simulink model "benchmark"  (R2024a)
settings: Solver=FixedStepAuto  StartTime=0.0  StopTime=10.0  FixedStep=0.001  RelTol=1e-3
InitFcn:
  | run("estimators_design.m")
libraries: cstblocks x1
settings Model: Creator=Bocchio  LastModifiedBy=Bocchio

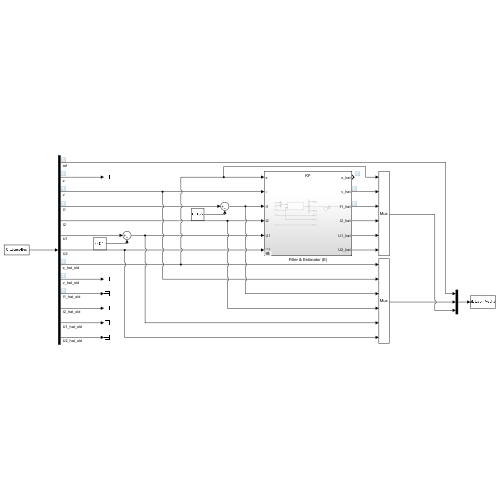
[thumbnail: Simulink's stored preview of the top-level diagram]
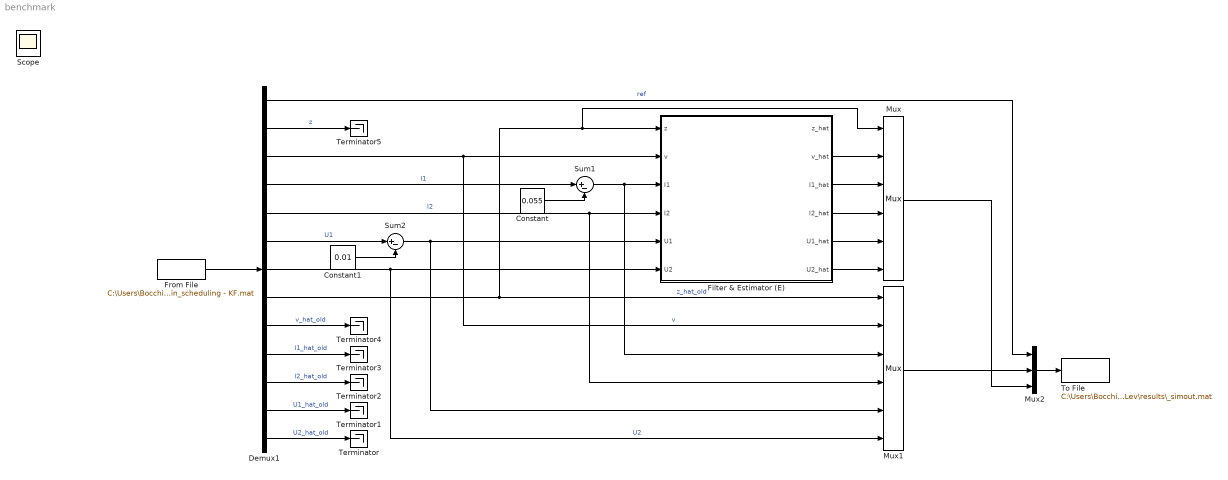
== system benchmark ==
  Constant : Constant  Value=0.055
  Constant1 : Constant  Value=0.01
  Demux1 : Demux  Outputs=13
  Filter & Estimator (E) : Subsystem  Variant=on  VariantControlMode=label  LabelModeActiveChoice=KF
  From File : FromFile  FileName=C:\Users\Bocchio\OneDrive\University\Lab - Mechatronics\MagLev\results\step\PID_gain_scheduling - KF.mat  SampleTime=0.001  InterpolationWithinTimeRange=Zero order hold
  Mux : Mux  Inputs=6
  Mux1 : Mux  Inputs=6
  Mux2 : Mux  Inputs=3
  Sum1 : Sum  Inputs=|+-
  Sum2 : Sum  Inputs=|+-
  Terminator{,1..5} (6 alike) : Terminator
  To File : ToFile  Filename=C:\Users\Bocchio\OneDrive\University\Lab - Mechatronics\MagLev\results\_simout.mat  MatrixName=logouts
  Scope : Scope
  wires:
  From File/1 -> Demux1/1
  Demux1/1 -> Mux2/1  "ref"
  Demux1/2 -> Terminator5/1  "z"
  Demux1/3 -> Mux1/2, Filter & Estimator (E)/2(v)  "v"
  Demux1/5 -> Mux1/4, Filter & Estimator (E)/4(I2)  "I2"
  Demux1/7 -> Filter & Estimator (E)/6(U2), Mux1/6  "U2"
  Demux1/8 -> Mux/1, Filter & Estimator (E)/1(z), Mux1/1  "z_hat_old"
  Demux1/9 -> Terminator4/1  "v_hat_old"
  Demux1/10 -> Terminator3/1  "I1_hat_old"
  Demux1/11 -> Terminator2/1  "I2_hat_old"
  Filter & Estimator (E)/2(v_hat) -> Mux/2
  Filter & Estimator (E)/3(I1_hat) -> Mux/3
  Filter & Estimator (E)/4(I2_hat) -> Mux/4
  Filter & Estimator (E)/5(U1_hat) -> Mux/5
  Filter & Estimator (E)/6(U2_hat) -> Mux/6
  Demux1/12 -> Terminator1/1  "U1_hat_old"
  Demux1/13 -> Terminator/1  "U2_hat_old"
  Mux/1 -> Mux2/3
  Mux2/1 -> To File/1
  Mux1/1 -> Mux2/2
  Constant/1 -> Sum1/2
  Demux1/4 -> Sum1/1  "I1"
  Sum1/1 -> Filter & Estimator (E)/3(I1), Mux1/3
  Constant1/1 -> Sum2/2
  Demux1/6 -> Sum2/1  "U1"
  Sum2/1 -> Mux1/5, Filter & Estimator (E)/5(U1)

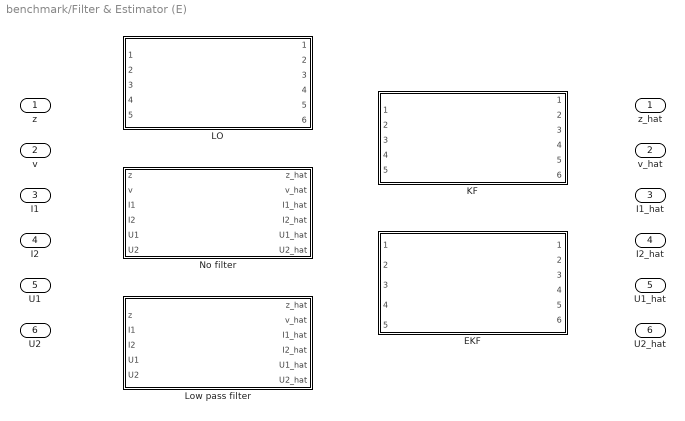
== system benchmark/Filter & Estimator (E) ==
  z : Inport
  v : Inport  Port=2
  I1 : Inport  Port=3
  I2 : Inport  Port=4
  U1 : Inport  Port=5
  U2 : Inport  Port=6
  EKF : Subsystem  VariantControl=EKF  ReferencedSubsystem=EKF
  KF : Subsystem  VariantControl=KF  ReferencedSubsystem=KF
  LO : Subsystem  VariantControl=LO  ReferencedSubsystem=LO
  Low pass filter : Subsystem  VariantControl=Low pass filter
  No filter : Subsystem  VariantControl=No filter
  z_hat : Outport
  v_hat : Outport  Port=2
  I1_hat : Outport  Port=3
  I2_hat : Outport  Port=4
  U1_hat : Outport  Port=5
  U2_hat : Outport  Port=6

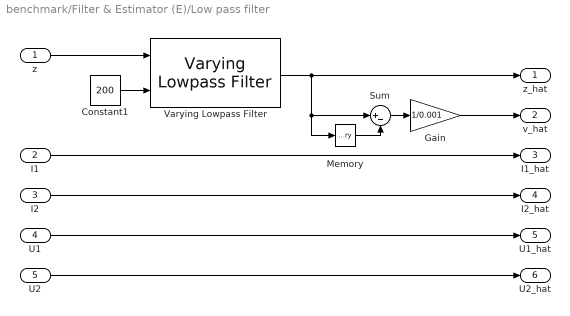
== system benchmark/Filter & Estimator (E)/Low pass filter ==
  z : Inport
  I1 : Inport  Port=2
  I2 : Inport  Port=3
  U1 : Inport  Port=4
  U2 : Inport  Port=5
  Constant1 : Constant  Value=200
  Gain : Gain  Gain=1/0.001
  Memory : Memory
  Sum : Sum  Inputs=|+-
  Varying Lowpass Filter : cstblocks/Linear Parameter Varying/Varying Lowpass Filter  N=1
  z_hat : Outport
  v_hat : Outport  Port=2
  I1_hat : Outport  Port=3
  I2_hat : Outport  Port=4
  U1_hat : Outport  Port=5
  U2_hat : Outport  Port=6
  wires:
  Constant1/1 -> Varying Lowpass Filter/2
  z/1 -> Varying Lowpass Filter/1
  Memory/1 -> Sum/2
  Sum/1 -> Gain/1
  U1/1 -> U1_hat/1
  Varying Lowpass Filter/1 -> Memory/1, Sum/1, z_hat/1
  U2/1 -> U2_hat/1
  Gain/1 -> v_hat/1
  I1/1 -> I1_hat/1
  I2/1 -> I2_hat/1

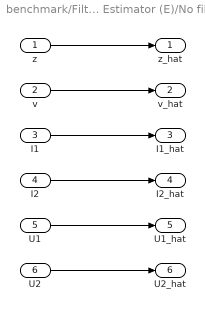
== system benchmark/Filter & Estimator (E)/No filter ==
  z : Inport
  v : Inport  Port=2
  I1 : Inport  Port=3
  I2 : Inport  Port=4
  U1 : Inport  Port=5
  U2 : Inport  Port=6
  z_hat : Outport
  v_hat : Outport  Port=2
  I1_hat : Outport  Port=3
  I2_hat : Outport  Port=4
  U1_hat : Outport  Port=5
  U2_hat : Outport  Port=6
  wires:
  z/1 -> z_hat/1
  v/1 -> v_hat/1
  I1/1 -> I1_hat/1
  I2/1 -> I2_hat/1
  U1/1 -> U1_hat/1
  U2/1 -> U2_hat/1
